simulink model "GSFR_based_on_Anderson_with_constant_Pd"  (R2019b)
settings: Solver=VariableStepAuto  StartTime=0  StopTime=20.0  MaxStep=0.01  RelTol=1e-3
model workspace (MAT data in the model file):
  H = [8 1]
libraries: dspsrcs4 x1
settings Model: EnablePacing=on  PacingRate=1000  ParameterArgumentNames=H  OrderedModelArguments=off  Creator=ruiva  LastModifiedBy=ruiva

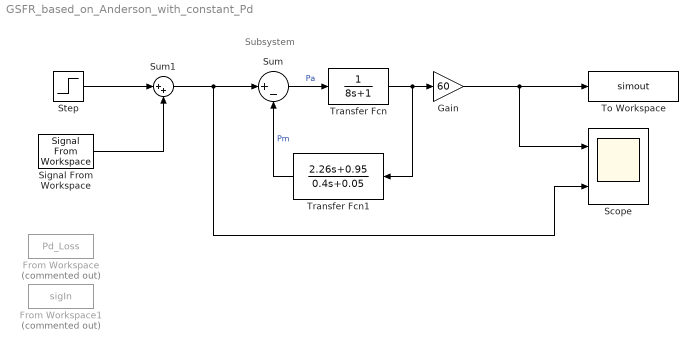
== system GSFR_based_on_Anderson_with_constant_Pd ==
  note: Subsystem
  From Workspace : FromWorkspace  Commented=on  VariableName=Pd_Loss  SampleTime=0
  From Workspace1 : FromWorkspace  Commented=on  VariableName=sigIn  SampleTime=0
  Gain : Gain  Gain=60
  Scope : Scope  NumInputPorts=2
  Signal From Workspace : dspsrcs4/Signal From Workspace  X=0:1  Ts=1  nsamps=1  OutputAfterFinalValue=Setting to zero  ignoreOrWarnInputAndFrameLengths=off  OutputFrames=off
  Step : Step  Time=0  After=-0.3  SampleTime=0  VectorParams1D=off  ZeroCross=off
  Sum : Sum  Inputs=|+-
  Sum1 : Sum  Inputs=|++
  To Workspace : ToWorkspace  VariableName=simout  SampleTime=-1
  Transfer Fcn : TransferFcn  Denominator=[8 1]
  Transfer Fcn1 : TransferFcn  Numerator=[2.26 0.95]  Denominator=[0.4 0.05]
  wires:
  Transfer Fcn1/1 -> Sum/2  "Pm"
  Transfer Fcn/1 -> Transfer Fcn1/1, Gain/1
  Gain/1 -> Scope/1, To Workspace/1
  Sum/1 -> Transfer Fcn/1  "Pa"
  Step/1 -> Sum1/1
  Sum1/1 -> Scope/2, Sum/1
  Signal From Workspace/1 -> Sum1/2
